simulink model "untitled"  (R2024a)
settings: Solver=VariableStepAuto  StartTime=0.0  StopTime=50  RelTol=1e-3
settings Model: Creator=Lenovo  LastModifiedBy=Lenovo

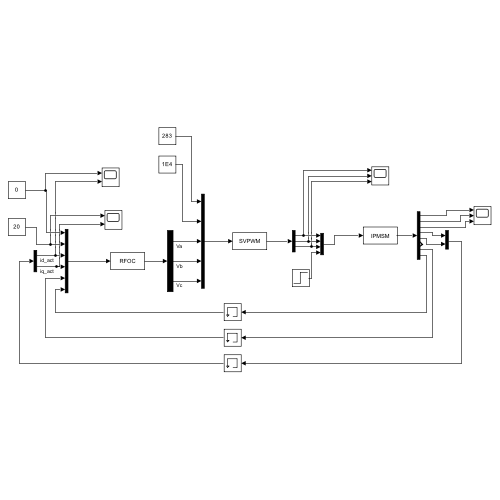
[thumbnail: Simulink's stored preview of the top-level diagram]
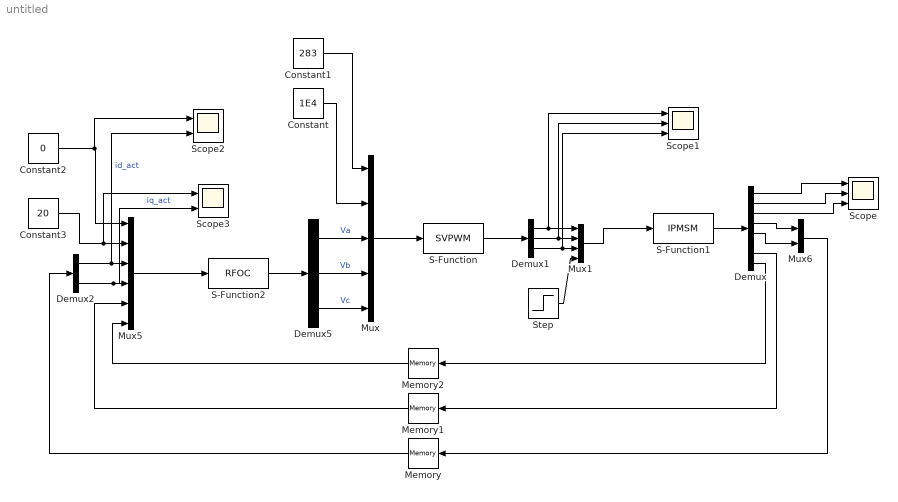
== system untitled ==
  Constant : Constant  Value=1E4
  Constant1 : Constant  Value=283
  Constant2 : Constant  Value=0
  Constant3 : Constant  Value=20
  Demux : Demux  Outputs=8
  Demux1 : Demux  Outputs=3
  Demux2 : Demux  Outputs=2
  Demux5 : Demux  Outputs=3
  Memory : Memory
  Memory1 : Memory
  Memory2 : Memory
  Mux : Mux  Inputs=5
  Mux1 : Mux
  Mux5 : Mux  Inputs=6
  Mux6 : Mux  Inputs=2
  S-Function : S-Function  FunctionName=SVPWM  SFunctionDeploymentMode=off  EnableBusSupport=off
  S-Function1 : S-Function  FunctionName=IPMSM  SFunctionDeploymentMode=off  EnableBusSupport=off
  S-Function2 : S-Function  FunctionName=RFOC  SFunctionDeploymentMode=off  EnableBusSupport=off
  Scope : Scope  NumInputPorts=3
  Scope1 : Scope  NumInputPorts=3
  Scope2 : Scope  NumInputPorts=2
  Scope3 : Scope  NumInputPorts=2
  Step : Step  After=0  SampleTime=0
  wires:
  Mux/1 -> S-Function/1
  Constant1/1 -> Mux/1
  Constant/1 -> Mux/2
  Demux/2 -> Scope/2
  Demux/3 -> Scope/3
  Demux/1 -> Scope/1
  S-Function1/1 -> Demux/1
  S-Function/1 -> Demux1/1
  Demux1/1 -> Scope1/1, Mux1/1
  Demux1/2 -> Scope1/2, Mux1/2
  Demux1/3 -> Scope1/3, Mux1/3
  Step/1 -> Mux1/4
  Mux1/1 -> S-Function1/1
  Mux5/1 -> S-Function2/1
  S-Function2/1 -> Demux5/1
  Demux5/1 -> Mux/3  "Va"
  Demux5/2 -> Mux/4  "Vb"
  Demux5/3 -> Mux/5  "Vc"
  Demux/4 -> Mux6/1
  Demux/5 -> Mux6/2
  Mux6/1 -> Memory/1
  Demux2/1 -> Scope2/2, Mux5/3  "id_act"
  Demux2/2 -> Scope3/2, Mux5/4  "iq_act"
  Memory/1 -> Demux2/1
  Constant2/1 -> Scope2/1, Mux5/1
  Constant3/1 -> Scope3/1, Mux5/2
  Demux/7 -> Memory1/1
  Demux/8 -> Memory2/1
  Memory1/1 -> Mux5/5
  Memory2/1 -> Mux5/6
